simulink model "TwoNxInterleavedBoostConverter_Ideal"  (R2018a)
settings: Solver=ode23tb  StartTime=0.0  StopTime=0.05  MaxStep=1e-6  RelTol=1e-3
libraries: powerlib x41, simulink x1
settings Model: Creator=Ilian  LastModifiedBy=Ilian
settings SolverCC: InitialStep=1e-8  ZeroCrossAlgorithm=Adaptive
settings DebuggingCC: MaxConsecutiveZCsMsg=none  MaskedZcDiagnostic=none  IgnoredZcDiagnostic=none  UnconnectedInputMsg=none  UnconnectedOutputMsg=none  UnconnectedLineMsg=none

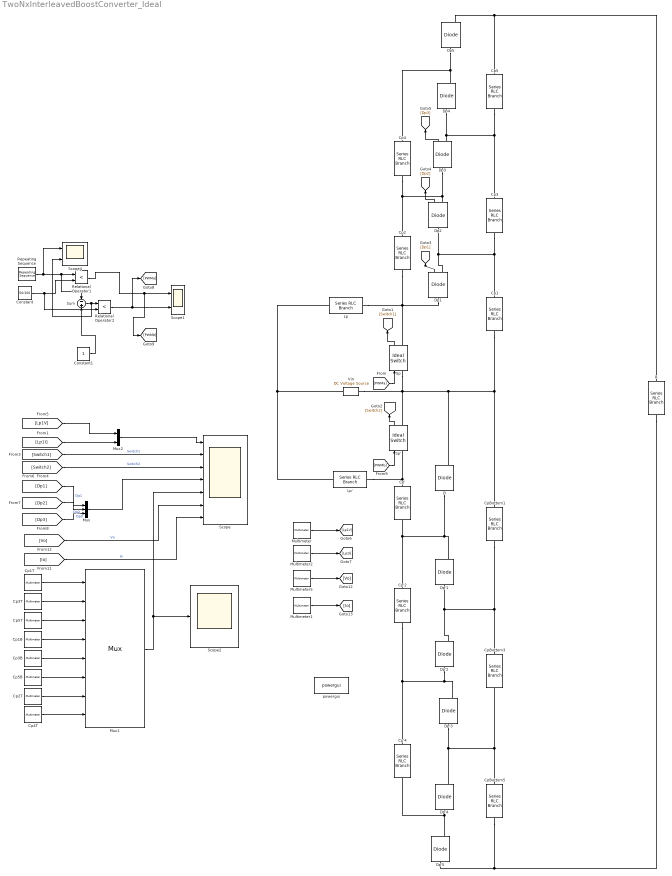
== system TwoNxInterleavedBoostConverter_Ideal ==
  "\tLp" : powerlib/Elements/Series RLC Branch  LConnTagsString=__new0  RConnTagsString=__new0  BranchType=L  Resistance=1  Inductance=150e-6  SetiL0=off  InitialCurrent=0  Capacitance=1e-6  Setx0=off  InitialVoltage=0  Measurements=Branch voltage and current
  "\tR" : powerlib/Elements/Series RLC Branch  LConnTagsString=__new0  RConnTagsString=__new0  BranchType=R  Resistance=225  Inductance=150e-6  SetiL0=off  InitialCurrent=0  Capacitance=1e-6  Setx0=off  InitialVoltage=0  Measurements=Branch voltage and current
  Constant : Constant  Value=50/100
  Constant1 : Constant
  Cp' : powerlib/Elements/Series RLC Branch  LConnTagsString=__new0  RConnTagsString=__new0  BranchType=C  Resistance=1  Inductance=150e-3  SetiL0=off  InitialCurrent=0  Capacitance=220e-6  Setx0=off  InitialVoltage=0  Measurements=None
  Cp'2 : powerlib/Elements/Series RLC Branch  LConnTagsString=__new0  RConnTagsString=__new0  BranchType=C  Resistance=1  Inductance=150e-3  SetiL0=off  InitialCurrent=0  Capacitance=220e-6  Setx0=off  InitialVoltage=0  Measurements=None
  Cp'4 : powerlib/Elements/Series RLC Branch  LConnTagsString=__new0  RConnTagsString=__new0  BranchType=C  Resistance=1  Inductance=150e-3  SetiL0=off  InitialCurrent=0  Capacitance=220e-6  Setx0=off  InitialVoltage=0  Measurements=None
  Cp{1..5} (5 alike) : powerlib/Elements/Series RLC Branch  LConnTagsString=__new0  RConnTagsString=__new0  BranchType=C  Resistance=1  Inductance=150e-3  SetiL0=off  InitialCurrent=0  Capacitance=220e-6  Setx0=off  InitialVoltage=0  Measurements=Branch voltage and current
  Cp1B : powerlib/Measurements/Multimeter  PhasorSimulation=off  OutputType=Complex  sel=8  L=19  Gain=1  yselected={'Ub: CpBottom1'};  PSBOutputType=1  PSBequivalent=0  AxesSetting=[0,0.1,-100,100]  Display=0  SavedBlockNames=-11
  Cp1T : powerlib/Measurements/Multimeter  PhasorSimulation=off  OutputType=Complex  sel=3  L=19  Gain=1  yselected={'Ub: Cp1'};  PSBOutputType=1  PSBequivalent=0  AxesSetting=[0,0.1,-100,100]  Display=0  SavedBlockNames=-11
  Cp2T : powerlib/Measurements/Multimeter  PhasorSimulation=off  OutputType=Complex  sel=4  L=19  Gain=1  yselected={'Ub: Cp2'};  PSBOutputType=1  PSBequivalent=0  AxesSetting=[0,0.1,-100,100]  Display=0  SavedBlockNames=-11
  Cp3B : powerlib/Measurements/Multimeter  PhasorSimulation=off  OutputType=Complex  sel=9  L=19  Gain=1  yselected={'Ub: CpBottom3'};  PSBOutputType=1  PSBequivalent=0  AxesSetting=[0,0.1,-100,100]  Display=0  SavedBlockNames=-11
  Cp3T : powerlib/Measurements/Multimeter  PhasorSimulation=off  OutputType=Complex  sel=5  L=19  Gain=1  yselected={'Ub: Cp3'};  PSBOutputType=1  PSBequivalent=0  AxesSetting=[0,0.1,-100,100]  Display=0  SavedBlockNames=-11
  Cp4T : powerlib/Measurements/Multimeter  PhasorSimulation=off  OutputType=Complex  sel=10  L=19  Gain=1  yselected={'Ub: CpBottom5'};  PSBOutputType=1  PSBequivalent=0  AxesSetting=[0,0.1,-100,100]  Display=0  SavedBlockNames=-11
  Cp5B : powerlib/Measurements/Multimeter  PhasorSimulation=off  OutputType=Complex  sel=10  L=19  Gain=1  yselected={'Ub: CpBottom5'};  PSBOutputType=1  PSBequivalent=0  AxesSetting=[0,0.1,-100,100]  Display=0  SavedBlockNames=-11
  Cp5T : powerlib/Measurements/Multimeter  PhasorSimulation=off  OutputType=Complex  sel=7  L=19  Gain=1  yselected={'Ub: Cp5'};  PSBOutputType=1  PSBequivalent=0  AxesSetting=[0,0.1,-100,100]  Display=0  SavedBlockNames=-11
  CpBottom1 : powerlib/Elements/Series RLC Branch  LConnTagsString=__new0  RConnTagsString=__new0  BranchType=C  Resistance=1  Inductance=150e-3  SetiL0=off  InitialCurrent=0  Capacitance=220e-6  Setx0=off  InitialVoltage=0  Measurements=Branch voltage
  CpBottom3 : powerlib/Elements/Series RLC Branch  LConnTagsString=__new0  RConnTagsString=__new0  BranchType=C  Resistance=1  Inductance=150e-3  SetiL0=off  InitialCurrent=0  Capacitance=220e-6  Setx0=off  InitialVoltage=0  Measurements=Branch voltage
  CpBottom5 : powerlib/Elements/Series RLC Branch  LConnTagsString=__new0  RConnTagsString=__new0  BranchType=C  Resistance=1  Inductance=150e-3  SetiL0=off  InitialCurrent=0  Capacitance=220e-6  Setx0=off  InitialVoltage=0  Measurements=Branch voltage
  D : powerlib/Power Electronics/Diode  Ron=0.001  Lon=0  Vf=0.8  IC=0  UseSnubber=0  Rs=500  Cs=250e-9  Measurements=on
  Dp'{1..5} (5 alike) : powerlib/Power Electronics/Diode  Ron=0.001  Lon=0  Vf=0.8  IC=0  UseSnubber=0  Rs=500  Cs=250e-9  Measurements=on
  Dp{1..5} (5 alike) : powerlib/Power Electronics/Diode  Ron=0.001  Lon=0  Vf=0.8  IC=0  UseSnubber=0  Rs=500  Cs=250e-9  Measurements=on
  Lp' : powerlib/Elements/Series RLC Branch  LConnTagsString=__new0  RConnTagsString=__new0  BranchType=L  Resistance=1  Inductance=150e-6  SetiL0=off  InitialCurrent=0  Capacitance=1e-6  Setx0=off  InitialVoltage=0  Measurements=Branch voltage and current
  Multimeter : powerlib/Measurements/Multimeter  PhasorSimulation=off  OutputType=Complex  sel=1  L=19  Gain=1  yselected="{'Ub: \tLp'};"  PSBOutputType=1  PSBequivalent=0  AxesSetting=[0,0.1,-100,100]  Display=0  SavedBlockNames=-11
  Multimeter1 : powerlib/Measurements/Multimeter  PhasorSimulation=off  OutputType=Complex  sel=13  L=19  Gain=1  yselected="{'Ib: \tR'};"  PSBOutputType=1  PSBequivalent=0  AxesSetting=[0,0.1,-100,100]  Display=0  SavedBlockNames=-11
  Multimeter2 : powerlib/Measurements/Multimeter  PhasorSimulation=off  OutputType=Complex  sel=1  L=19  Gain=1  yselected="{'Ub: \tLp'};"  PSBOutputType=1  PSBequivalent=0  AxesSetting=[0,0.1,-100,100]  Display=0  SavedBlockNames=-11
  Multimeter5 : powerlib/Measurements/Multimeter  PhasorSimulation=off  OutputType=Complex  sel=2  L=19  Gain=1  yselected="{'Ub: \tR'};"  PSBOutputType=1  PSBequivalent=0  AxesSetting=[0,0.1,-100,100]  Display=0  SavedBlockNames=-11
  Mux : Mux  Inputs=3
  Mux1 : Mux  Inputs=8
  Mux2 : Mux  Inputs=2
  Relational Operator1 : RelationalOperator  Operator=<  OutDataTypeStr=boolean  RndMeth=Simplest
  Relational Operator2 : RelationalOperator  Operator=<  OutDataTypeStr=boolean  RndMeth=Simplest
  Repeating Sequence : simulink/Sources/Repeating Sequence  rep_seq_t=[0 1/2 1]*(1/50000)  rep_seq_y=[0 1 0]
  Scope : Scope  NumInputPorts=7
  Scope1 : Scope  NumInputPorts=2
  Scope2 : Scope
  Scope4 : Scope  NumInputPorts=2
  Sp : powerlib/Power Electronics/Ideal Switch  Ron=0.001  Lon=0  IC=0  Rs=1e5  Cs=inf  Measurements=on
  Sp' : powerlib/Power Electronics/Ideal Switch  Ron=0.001  Lon=0  IC=0  Rs=1e5  Cs=inf  Measurements=on
  Sum : Sum  Inputs=-+
  Vin : powerlib/Electrical Sources/DC Voltage Source  Amplitude=10  Measurements=None
  powergui : powerlib/powergui  Priority=1  SimulationMode=Continuous  SampleTime=50e-6  frequency=60  Iterations=50  frequencyindice=0  Pbase=100e6  ErrMax=1e-4  UnitsV=kV  UnitsW=MW  buscounter=0  FunctionMessages=off  echomessages=off  EnableUseOfTLC=off  CurrentSourceSwitches=off  DisableSnubberDevices=off  DisableRonSwitches=off  DisableVfSwitches=off  DisplayEquations=off  SolverType=Tustin/Backward Euler (TBE)  Interpol=off  ExternalGateDelay=off  methode=off  Ts=100  x0status=blocks  SPID=on  SwTol=0  HookPort=off  RestoreLinks=warning  ResistiveCurrentMeasurement=off  Frange=[0:2:500]  Ylog=off  Xlog=on  ShowGrid=off  save=off  variable=ZData  structure=0  ZoomFFT=off  StartTime=0.0  cycles=1  DisplayStyle=1  fundamental=60  FreqAxis=off  MaxFrequency=1000  frequencyindicesteady=1  RmsSteady=1  display=off
  wires:
  Relational Operator2/1 -> [PWMa], Scope1/2
  Constant1/1 -> Sum/2
  Sum/1 -> Scope4/2, Relational Operator2/1
  Constant/1 -> Relational Operator2/2, Relational Operator1/2
  Repeating Sequence/1 -> Scope4/1, Sum/1, Relational Operator1/1
  Relational Operator1/1 -> [PWMb], Scope1/1
  [PWMa] -> Sp/1
  [PWMb] -> Sp'/1
  Sp/1 -> [Switch1]
  Sp'/1 -> [Switch2]
  [Switch1] -> Scope/2  "Switch1"
  Dp1/1 -> [Dp1]
  Dp2/1 -> [Dp2]
  Dp3/1 -> [Dp3]
  Multimeter/1 -> [Lp1V]
  [Switch2] -> Scope/3  "Swtich2"
  [Dp1] -> Mux/1  "Dp1"
  [Dp2] -> Mux/2  "Dp2"
  [Dp3] -> Mux/3  "Dp3"
  Mux/1 -> Scope/4
  Multimeter5/1 -> [Vo]
  [Vo] -> Scope/6  "Vo"
  Multimeter1/1 -> [Io]
  [Io] -> Scope/7  "Io"
  Cp1T/1 -> Mux1/1
  Cp3T/1 -> Mux1/2
  Cp5T/1 -> Mux1/3
  Cp1B/1 -> Mux1/4
  Cp3B/1 -> Mux1/5
  Cp5B/1 -> Mux1/6
  Cp2T/1 -> Mux1/7
  Cp4T/1 -> Mux1/8
  Multimeter2/1 -> [Lp1I]
  [Lp1V] -> Mux2/1
  [Lp1I] -> Mux2/2
  Mux2/1 -> Scope/1
  Mux1/1 -> Scope2/1, Scope/5
  connections:
  Vin/RConn1 -- Lp'/LConn1 -- "\tLp"/LConn1
  "\tLp"/RConn1 -- Cp2/RConn1 -- Dp1/LConn1 -- Sp/RConn1
  CpBottom1/LConn1 -- Sp/LConn1 -- Sp'/RConn1 -- Vin/LConn1 -- D/RConn1 -- Cp1/RConn1
  Lp'/RConn1 -- Sp'/LConn1 -- Cp'/LConn1
  Cp3/RConn1 -- Dp1/RConn1 -- Dp2/LConn1 -- Cp1/LConn1
  Dp2/RConn1 -- Cp4/RConn1 -- Cp2/LConn1 -- Dp3/LConn1
  Cp3/LConn1 -- Cp5/RConn1 -- Dp4/LConn1 -- Dp3/RConn1
  CpBottom1/RConn1 -- Dp'2/RConn1 -- Dp'1/LConn1 -- CpBottom3/LConn1
  Dp'1/RConn1 -- D/LConn1 -- Cp'2/LConn1 -- Cp'/RConn1
  Dp'2/LConn1 -- Cp'4/LConn1 -- Cp'2/RConn1 -- Dp'3/RConn1
  Dp'3/LConn1 -- Dp'4/RConn1 -- CpBottom5/LConn1 -- CpBottom3/RConn1
  Cp4/LConn1 -- Dp5/LConn1 -- Dp4/RConn1
  Dp'4/LConn1 -- Dp'5/RConn1 -- Cp'4/RConn1
  CpBottom5/RConn1 -- "\tR"/RConn1 -- Dp'5/LConn1
  Dp5/RConn1 -- Cp5/LConn1 -- "\tR"/LConn1
